simulink model "test"  (R2018b)
settings: Solver=VariableStepAuto  StartTime=0.0  StopTime=10.0  MaxStep=0.1  RelTol=1e-3
settings Model: Creator=kekos  LastModifiedBy=kekos

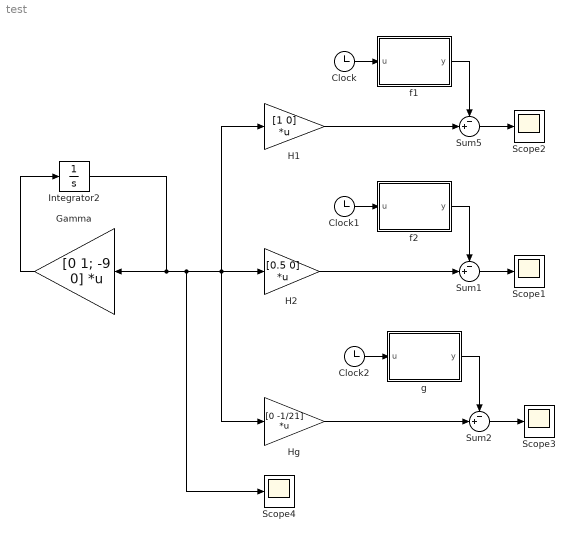
== system test ==
  Clock : Clock
  Clock1 : Clock
  Clock2 : Clock
  Gamma : Gain  Gain=[0 1; -9 0]  Multiplication=Matrix(K*u)
  H1 : Gain  Gain=[1 0]  Multiplication=Matrix(K*u)
  H2 : Gain  Gain=[0.5 0]  Multiplication=Matrix(K*u)
  Hg : Gain  Gain=[0 -1/21]  Multiplication=Matrix(K*u)
  Integrator2 : Integrator  InitialCondition=[-2.91; -19.10]
  Scope{1..4} (4 alike) : Scope
  Sum1 : Sum  Inputs=-+|
  Sum2 : Sum  Inputs=-+|
  Sum5 : Sum  Inputs=-+|
  f1 : MATLAB Function  TreatAsAtomicUnit=on
  f2 : MATLAB Function  TreatAsAtomicUnit=on
  g : MATLAB Function  TreatAsAtomicUnit=on
  wires:
  Gamma/1 -> Integrator2/1
  Integrator2/1 -> Scope4/1, H1/1, H2/1, Hg/1, Gamma/1
  Sum5/1 -> Scope2/1
  Clock/1 -> f1/1(u)
  H1/1 -> Sum5/2
  f1/1(y) -> Sum5/1
  f2/1(y) -> Sum1/1
  H2/1 -> Sum1/2
  Sum1/1 -> Scope1/1
  Clock1/1 -> f2/1(u)
  g/1(y) -> Sum2/1
  Hg/1 -> Sum2/2
  Sum2/1 -> Scope3/1
  Clock2/1 -> g/1(u)

== matlab function test/f2 ==
  data: u input; y output
function y = fcn(u)

y = 3.5*cos(3*u+2);

== matlab function test/f1 ==
  data: u input; y output
function y = fcn(u)

y = 7*cos(3*u+2);

== matlab function test/g ==
  data: u input; y output
function y = fcn(u)

y = sin(3*u+2);
